simulink model "BolandLab5"  (R2024b)
settings: Solver=ode15s  StartTime=0.0  StopTime=100  RelTol=1e-3
settings Model: Creator=localdmluser  LastModifiedBy=localdmluser

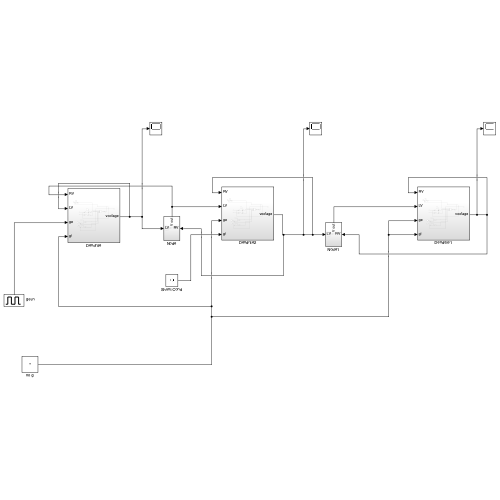
[thumbnail: Simulink's stored preview of the top-level diagram]
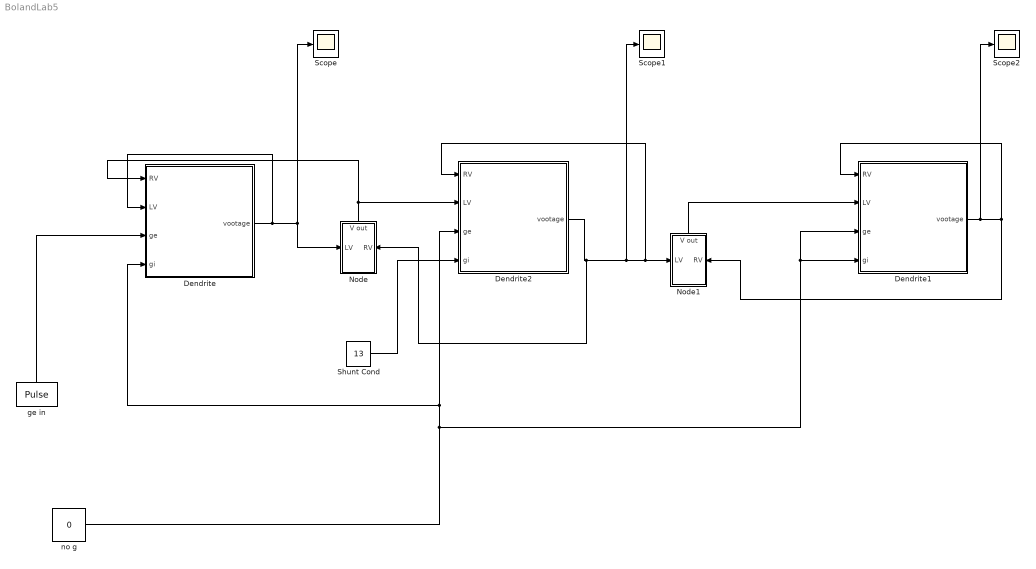
== system BolandLab5 ==
  Dendrite : Subsystem
  Dendrite1 : Subsystem
  Dendrite2 : Subsystem
  Node : Subsystem
      settings: PortSchema="{\"entries\":[{\"content\":{\"sides\":[{\"content\":{\"connectorIds\":[\"In1\"]},\"type\":\"ConnectorPlacement.EquallySpacedRectSide\",\"uuid\":\"358421d7-00fa-4f1a-ba9f-0ceb3a827095\"},{\"content\":{\"connectorIds\":[\"In2\"],\"side\":\"RIGHT\"},\"type\":\"ConnectorPlacement.EquallySpacedRectSide\",\"uuid\":\"7e4aef57-ce67-4e21-bc22-bec7d1c76f25\"},{\"content\":{\"connectorIds\":[\"Out1\"],\"side\":\"TOP\"},\"type\":\"ConnectorPlacement.EquallySpacedRectSide\",\"uuid\":\"d8bb780d-bc4c-49c5-9f36-4306442d6c64\"}]},\"type\":\"ConnectorPlacement.EquallySpacedConnector\",\"uuid\":\"198a5a76-6489-40e1-804d-f2b4860edd3e\"}],\"packageUris\":[\"http://schema.mathworks.com/mf0/Connector/R2020b\"],\"version\":\"1.0\"}"
  Node1 : Subsystem
      settings: PortSchema="{\"entries\":[{\"content\":{\"sides\":[{\"content\":{\"connectorIds\":[\"In1\"]},\"type\":\"ConnectorPlacement.EquallySpacedRectSide\",\"uuid\":\"358421d7-00fa-4f1a-ba9f-0ceb3a827095\"},{\"content\":{\"connectorIds\":[\"In2\"],\"side\":\"RIGHT\"},\"type\":\"ConnectorPlacement.EquallySpacedRectSide\",\"uuid\":\"7e4aef57-ce67-4e21-bc22-bec7d1c76f25\"},{\"content\":{\"connectorIds\":[\"Out1\"],\"side\":\"TOP\"},\"type\":\"ConnectorPlacement.EquallySpacedRectSide\",\"uuid\":\"d8bb780d-bc4c-49c5-9f36-4306442d6c64\"}]},\"type\":\"ConnectorPlacement.EquallySpacedConnector\",\"uuid\":\"198a5a76-6489-40e1-804d-f2b4860edd3e\"}],\"packageUris\":[\"http://schema.mathworks.com/mf0/Connector/R2020b\"],\"version\":\"1.0\"}"
  Scope : Scope
  Scope1 : Scope
  Scope2 : Scope
  Shunt Cond : Constant  Value=13
  ge in : DiscretePulseGenerator  PulseType=Time based  Amplitude=1.3  Period=100  PulseWidth=10
  no g : Constant  Value=0
  wires:
  Dendrite/1(vootage) -> Dendrite/2(LV), Scope/1, Node/1(LV)
  Dendrite2/1(vootage) -> Scope1/1, Dendrite2/1(RV), Node1/1(LV), Node/2(RV)
  Dendrite1/1(vootage) -> Dendrite1/1(RV), Node1/2(RV), Scope2/1
  Node1/1(V out) -> Dendrite1/2(LV)
  Node/1(V out) -> Dendrite/1(RV), Dendrite2/2(LV)
  no g/1 -> Dendrite1/4(gi), Dendrite1/3(ge), Dendrite/4(gi), Dendrite2/3(ge)
  ge in/1 -> Dendrite/3(ge)
  Shunt Cond/1 -> Dendrite2/4(gi)

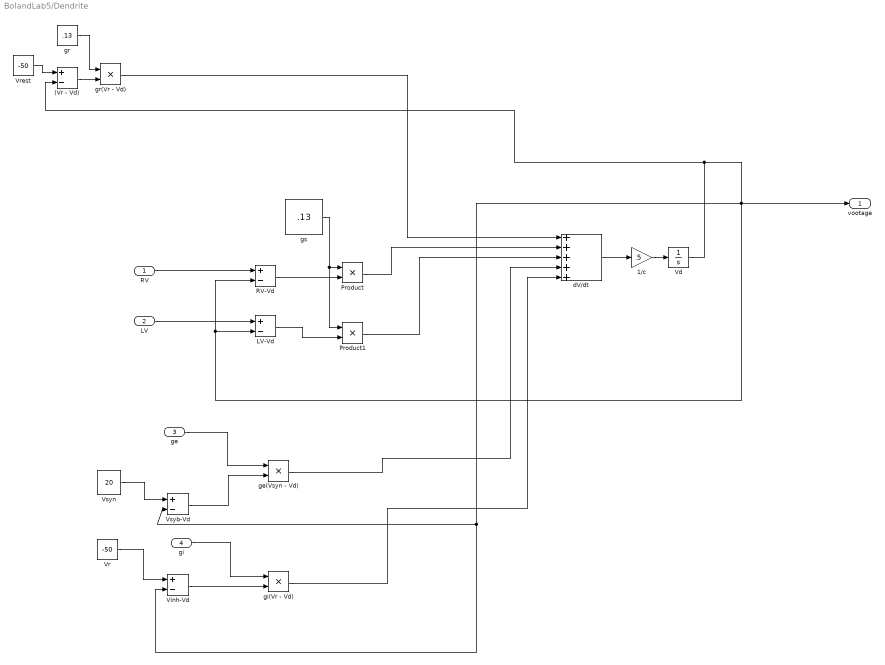
== system BolandLab5/Dendrite ==
  RV : Inport
  LV : Inport  Port=2
  ge : Inport  Port=3
  gi : Inport  Port=4
  (Vr - Vd) : Sum  Inputs=+-
  1/c : Gain  Gain=.5
  LV-Vd : Sum  Inputs=+-
  Product : Product
  Product1 : Product
  RV-Vd : Sum  Inputs=+-
  Vd : Integrator  InitialCondition=-50
  Vinh-Vd : Sum  Inputs=+-
  Vr : Constant  Value=-50
  Vrest : Constant  Value=-50
  Vsyb-Vd : Sum  Inputs=+-
  Vsyn : Constant  Value=20
  dV/dt : Sum  Inputs=+++++
  ge(Vsyn - Vd) : Product
  gi(Vr - Vd) : Product
  gr : Constant  Value=.13
  gr(Vr - Vd) : Product
  gs : Constant  Value=.13
  vootage : Outport
  wires:
  Vrest/1 -> (Vr - Vd)/1
  Vsyn/1 -> Vsyb-Vd/1
  RV-Vd/1 -> Product/2
  gs/1 -> Product1/1, Product/1
  LV/1 -> LV-Vd/1
  Vr/1 -> Vinh-Vd/1
  Vinh-Vd/1 -> gi(Vr - Vd)/2
  LV-Vd/1 -> Product1/2
  Vsyb-Vd/1 -> ge(Vsyn - Vd)/2
  dV/dt/1 -> 1/c/1
  gr(Vr - Vd)/1 -> dV/dt/1
  (Vr - Vd)/1 -> gr(Vr - Vd)/2
  ge(Vsyn - Vd)/1 -> dV/dt/4
  Product/1 -> dV/dt/2
  Product1/1 -> dV/dt/3
  gr/1 -> gr(Vr - Vd)/1
  RV/1 -> RV-Vd/1
  gi(Vr - Vd)/1 -> dV/dt/5
  gi/1 -> gi(Vr - Vd)/1
  Vd/1 -> (Vr - Vd)/2, RV-Vd/2, LV-Vd/2, vootage/1, Vinh-Vd/2, Vsyb-Vd/2
  1/c/1 -> Vd/1
  ge/1 -> ge(Vsyn - Vd)/1

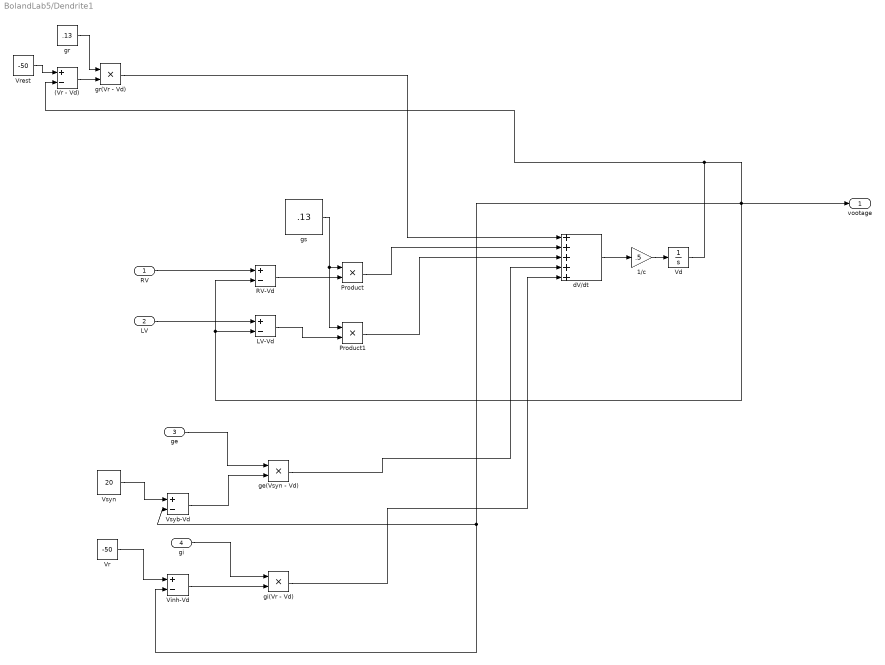
== system BolandLab5/Dendrite1 ==
  RV : Inport
  LV : Inport  Port=2
  ge : Inport  Port=3
  gi : Inport  Port=4
  (Vr - Vd) : Sum  Inputs=+-
  1/c : Gain  Gain=.5
  LV-Vd : Sum  Inputs=+-
  Product : Product
  Product1 : Product
  RV-Vd : Sum  Inputs=+-
  Vd : Integrator  InitialCondition=-50
  Vinh-Vd : Sum  Inputs=+-
  Vr : Constant  Value=-50
  Vrest : Constant  Value=-50
  Vsyb-Vd : Sum  Inputs=+-
  Vsyn : Constant  Value=20
  dV/dt : Sum  Inputs=+++++
  ge(Vsyn - Vd) : Product
  gi(Vr - Vd) : Product
  gr : Constant  Value=.13
  gr(Vr - Vd) : Product
  gs : Constant  Value=.13
  vootage : Outport
  wires:
  Vrest/1 -> (Vr - Vd)/1
  Vsyn/1 -> Vsyb-Vd/1
  RV-Vd/1 -> Product/2
  gs/1 -> Product1/1, Product/1
  LV/1 -> LV-Vd/1
  Vr/1 -> Vinh-Vd/1
  Vinh-Vd/1 -> gi(Vr - Vd)/2
  LV-Vd/1 -> Product1/2
  Vsyb-Vd/1 -> ge(Vsyn - Vd)/2
  dV/dt/1 -> 1/c/1
  gr(Vr - Vd)/1 -> dV/dt/1
  (Vr - Vd)/1 -> gr(Vr - Vd)/2
  ge(Vsyn - Vd)/1 -> dV/dt/4
  Product/1 -> dV/dt/2
  Product1/1 -> dV/dt/3
  gr/1 -> gr(Vr - Vd)/1
  RV/1 -> RV-Vd/1
  gi(Vr - Vd)/1 -> dV/dt/5
  gi/1 -> gi(Vr - Vd)/1
  Vd/1 -> (Vr - Vd)/2, RV-Vd/2, LV-Vd/2, vootage/1, Vinh-Vd/2, Vsyb-Vd/2
  1/c/1 -> Vd/1
  ge/1 -> ge(Vsyn - Vd)/1

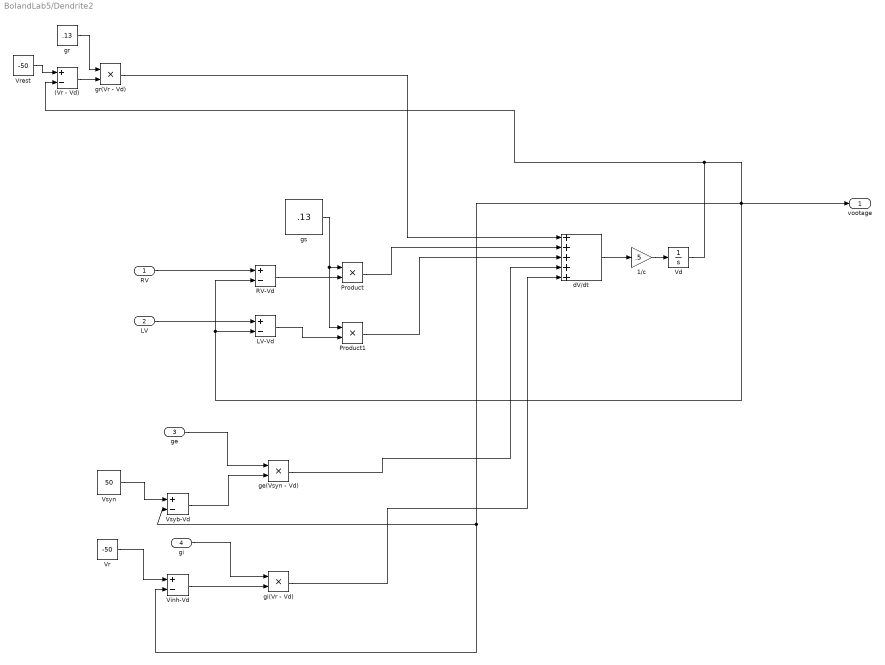
== system BolandLab5/Dendrite2 ==
  RV : Inport
  LV : Inport  Port=2
  ge : Inport  Port=3
  gi : Inport  Port=4
  (Vr - Vd) : Sum  Inputs=+-
  1/c : Gain  Gain=.5
  LV-Vd : Sum  Inputs=+-
  Product : Product
  Product1 : Product
  RV-Vd : Sum  Inputs=+-
  Vd : Integrator  InitialCondition=-50
  Vinh-Vd : Sum  Inputs=+-
  Vr : Constant  Value=-50
  Vrest : Constant  Value=-50
  Vsyb-Vd : Sum  Inputs=+-
  Vsyn : Constant  Value=50
  dV/dt : Sum  Inputs=+++++
  ge(Vsyn - Vd) : Product
  gi(Vr - Vd) : Product
  gr : Constant  Value=.13
  gr(Vr - Vd) : Product
  gs : Constant  Value=.13
  vootage : Outport
  wires:
  ge/1 -> ge(Vsyn - Vd)/1
  1/c/1 -> Vd/1
  Vd/1 -> Vsyb-Vd/2, Vinh-Vd/2, vootage/1, LV-Vd/2, RV-Vd/2, (Vr - Vd)/2
  gi/1 -> gi(Vr - Vd)/1
  gi(Vr - Vd)/1 -> dV/dt/5
  RV/1 -> RV-Vd/1
  gr/1 -> gr(Vr - Vd)/1
  Product1/1 -> dV/dt/3
  Product/1 -> dV/dt/2
  ge(Vsyn - Vd)/1 -> dV/dt/4
  (Vr - Vd)/1 -> gr(Vr - Vd)/2
  gr(Vr - Vd)/1 -> dV/dt/1
  dV/dt/1 -> 1/c/1
  Vsyb-Vd/1 -> ge(Vsyn - Vd)/2
  LV-Vd/1 -> Product1/2
  Vinh-Vd/1 -> gi(Vr - Vd)/2
  Vr/1 -> Vinh-Vd/1
  LV/1 -> LV-Vd/1
  gs/1 -> Product/1, Product1/1
  RV-Vd/1 -> Product/2
  Vsyn/1 -> Vsyb-Vd/1
  Vrest/1 -> (Vr - Vd)/1

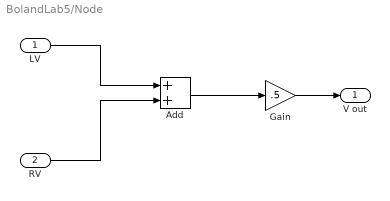
== system BolandLab5/Node ==
  LV : Inport
  RV : Inport  Port=2
  Add : Sum
  Gain : Gain  Gain=.5
  V out : Outport
  wires:
  LV/1 -> Add/1
  Gain/1 -> V out/1
  Add/1 -> Gain/1
  RV/1 -> Add/2

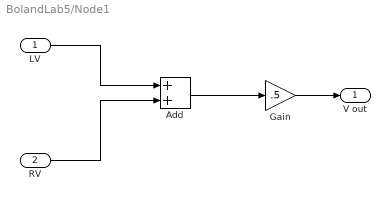
== system BolandLab5/Node1 ==
  LV : Inport
  RV : Inport  Port=2
  Add : Sum
  Gain : Gain  Gain=.5
  V out : Outport
  wires:
  LV/1 -> Add/1
  Gain/1 -> V out/1
  Add/1 -> Gain/1
  RV/1 -> Add/2
